simulink model "Stoppuhr"  (R2021b)
settings: Solver=ode3  StartTime=0.0  StopTime=10.0  FixedStep=0.01  RelTol=1e-3
libraries: simulink x1
settings Model: Creator=mwjae  LastModifiedBy=mwjae

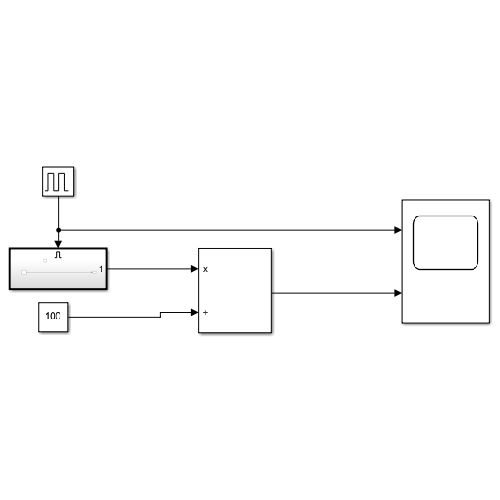
[thumbnail: Simulink's stored preview of the top-level diagram]
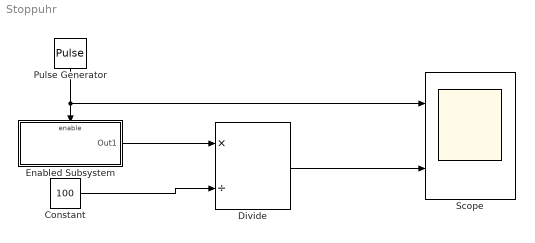
== system Stoppuhr ==
  Constant : Constant  Value=100
  Divide : Product  Inputs=*/
  Enabled Subsystem : Subsystem  TreatAsAtomicUnit=on
  Pulse Generator : DiscretePulseGenerator  PulseType=Time based  PulseWidth=50
  Scope : Scope  NumInputPorts=2
  wires:
  Pulse Generator/1 -> Enabled Subsystem/Enable, Scope/1
  Constant/1 -> Divide/2
  Enabled Subsystem/1(Out1) -> Divide/1
  Divide/1 -> Scope/2

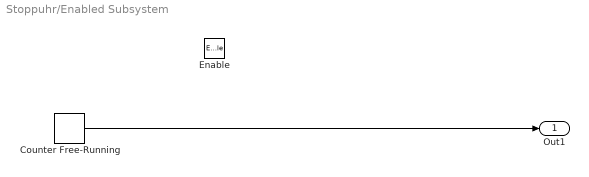
== system Stoppuhr/Enabled Subsystem ==
  Enable : EnablePort
  Counter Free-Running : simulink/Sources/Counter Free-Running  NumBits=16  tsamp=-1
  Out1 : Outport
  wires:
  Counter Free-Running/1 -> Out1/1
